simulink model "lab4_wtf"  (Simulink 6.6)
settings: Solver=ode45  StartTime=0.0  StopTime=100  RelTol=1e-3
settings Model: Creator=student  LastModifiedBy=student

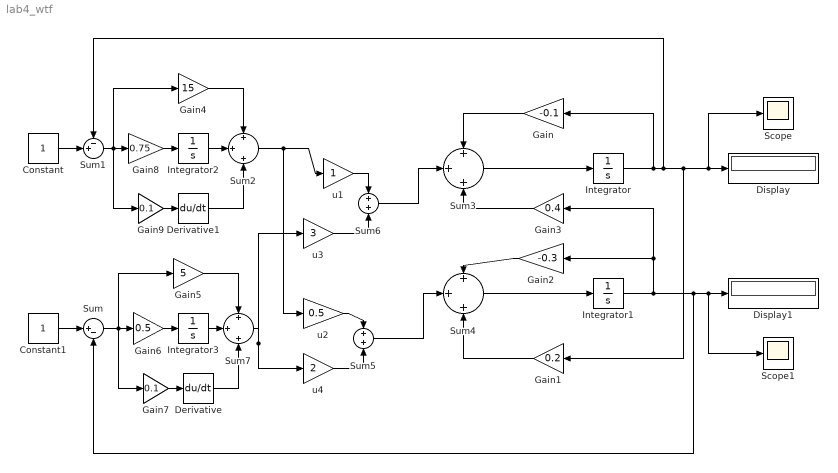
== system lab4_wtf ==
  Constant : Constant
  Constant1 : Constant
  Derivative : Derivative
  Derivative1 : Derivative
  Display : Display
  Display1 : Display
  Gain : Gain  Orientation=left  Gain=-0.1
  Gain1 : Gain  Orientation=left  Gain=0.2
  Gain2 : Gain  Orientation=left  Gain=-0.3
  Gain3 : Gain  Orientation=left  Gain=0.4
  Gain4 : Gain  Gain=15
  Gain5 : Gain  Gain=5
  Gain6 : Gain  Gain=0.5
  Gain7 : Gain  Gain=0.1
  Gain8 : Gain  Gain=0.75
  Gain9 : Gain  Gain=0.1
  Integrator{,1..3} (4 alike) : Integrator
  Scope : Scope
      settings: YMin=-0.00079  YMax=-0.00061
  Scope1 : Scope
  Sum : Sum  Inputs=|+-
  Sum1 : Sum  Inputs=-+|
  Sum{2..4,7} (4 alike) : Sum  Inputs=+|+|+
  Sum5 : Sum  Inputs=+|+
  Sum6 : Sum  Inputs=+|+
  u1 : Gain
  u2 : Gain  Gain=0.5
  u3 : Gain  Gain=3
  u4 : Gain  Gain=2
  wires:
  Sum/1 -> Gain5/1, Gain6/1, Gain7/1
  Constant1/1 -> Sum/1
  Sum1/1 -> Gain4/1, Gain8/1, Gain9/1
  Constant/1 -> Sum1/2
  Sum3/1 -> Integrator/1
  Sum4/1 -> Integrator1/1
  Integrator/1 -> Gain/1, Gain1/1, Display/1, Scope/1, Sum1/1
  Gain/1 -> Sum3/1
  Integrator1/1 -> Gain2/1, Gain3/1, Sum/2, Display1/1, Scope1/1
  Gain3/1 -> Sum3/3
  Gain2/1 -> Sum4/1
  Gain1/1 -> Sum4/3
  u1/1 -> Sum6/1
  u3/1 -> Sum6/2
  u2/1 -> Sum5/1
  u4/1 -> Sum5/2
  Sum6/1 -> Sum3/2
  Sum5/1 -> Sum4/2
  Integrator2/1 -> Sum2/2
  Gain4/1 -> Sum2/1
  Integrator3/1 -> Sum7/2
  Gain5/1 -> Sum7/1
  Gain6/1 -> Integrator3/1
  Gain7/1 -> Derivative/1
  Derivative/1 -> Sum7/3
  Gain8/1 -> Integrator2/1
  Gain9/1 -> Derivative1/1
  Derivative1/1 -> Sum2/3
  Sum2/1 -> u1/1, u2/1
  Sum7/1 -> u4/1, u3/1
